simulink model "a_sim_1"  (R2020a)
settings: Solver=VariableStepAuto  StartTime=0.0  StopTime=10.0  RelTol=1e-3
values from neighbouring files (symbols this model uses):
  buffer = 0.0    (= 0)    [a_1.m]    (also in a_2.m; a_loss_function.m; full_model.m; part2.m)
  c_fi = 0.5    [a_1.m]    (also in a_2.m; a_loss_function.m; bank_and_economy.m = 0.25)
  gov = 0.5    [a_1.m]    (also in a_2.m; a_loss_function.m; bank_centralbank.m; full_model.m)
  hike = 0.0    (= 0)    [a_1.m]    (also in a_2.m = 0.01; a_loss_function.m; full_model.m; part2.m = 0.01)
  i_cb = 0.03    [a_1.m]    (also in a_2.m = 0.07; a_loss_function.m; full_model.m; part2.m = 0.1)
  i_diff = 0.025    [a_1.m]    (also in a_2.m; a_loss_function.m; bank_and_economy.m = 0.02; full_model.m)
  i_k = 0.06    [a_1.m]    (also in a_loss_function.m = 0.04; bank_and_economy.m = 0.04; full_model.m = 0.04)
  K_p = 15    [a_1.m]    (also in a_2.m; a_loss_function.m; bank_and_economy.m = 0.5; bank_centralbank.m)
  lambda = 0.002    [a_1.m]    (also in a_2.m; a_loss_function.m; bank_and_economy.m; bank_centralbank.m)
  lambda_k = 0.005    [a_1.m]    (also in a_2.m; a_loss_function.m; full_model.m; part2.m)
  R = 1    [a_1.m]    (also in a_2.m; a_loss_function.m; bank_and_economy.m; bank_centralbank.m)
  r_k = 0.1    [a_1.m]    (also in a_2.m; a_loss_function.m; bank_and_economy.m; full_model.m)
  rate = 0.1    [a_1.m]    (also in a_2.m; a_loss_function.m; bank_and_economy.m; bank_centralbank.m)
  s_k = 0.25    [a_1.m]    (also in a_2.m; bank_and_economy.m; part2.m = 0.2; part_1.m = 0.2)
  sigma = 0.28    [a_1.m]    (also in a_2.m; a_loss_function.m; bank_and_economy.m; bank_centralbank.m)
  T_f = 0.5    [a_1.m]    (also in a_2.m; a_loss_function.m; bank_and_economy.m; bank_centralbank.m)
  T_g = 1    [a_1.m]    (also in a_2.m; a_loss_function.m; bank_and_economy.m; bank_centralbank.m)
  T_h = 0.1    [a_1.m]    (also in a_2.m; a_loss_function.m; bank_and_economy.m; bank_centralbank.m)
  T_i = 8    [a_1.m]    (also in a_2.m; a_loss_function.m; bank_and_economy.m; bank_centralbank.m)
  T_k = 0.1    [a_1.m]    (also in a_2.m; a_loss_function.m; bank_and_economy.m = 0.25; economy.m = 1)
  tx = 0.3    [a_1.m]    (also in a_2.m; a_loss_function.m; bank_and_economy.m = 0.5; bank_centralbank.m = 0.25)
settings Model: Creator=erlended  LastModifiedBy=erlended

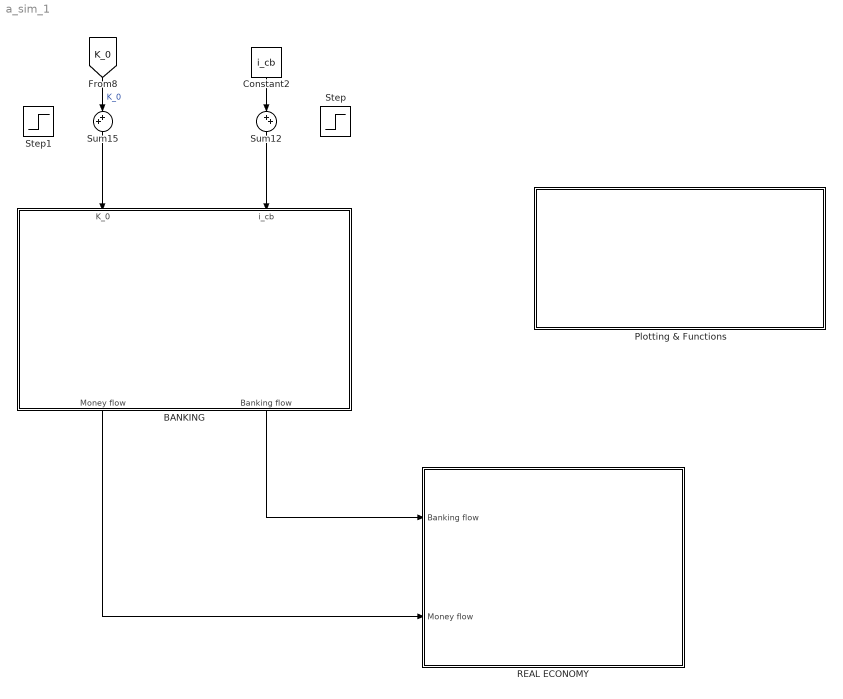
== system a_sim_1 ==
  BANKING : Subsystem
  Constant2 : Constant  Value=i_cb
  Plotting & Functions : Subsystem
  REAL ECONOMY : Subsystem
  Step : Step  Time=10  After=hike  SampleTime=0
  Step1 : Step  Time=10  After=buffer  SampleTime=0
  Sum12 : Sum  Inputs=|++
  Sum15 : Sum  Inputs=++|
  wires:
  Constant2/1 -> Sum12/1
  [K_0] -> Sum15/2  "K_0"
  BANKING/2(Banking flow) -> REAL ECONOMY/1(Banking flow)
  Sum12/1 -> BANKING/2(i_cb)
  BANKING/1(Money flow) -> REAL ECONOMY/2(Money flow)
  Sum15/1 -> BANKING/1(K_0)

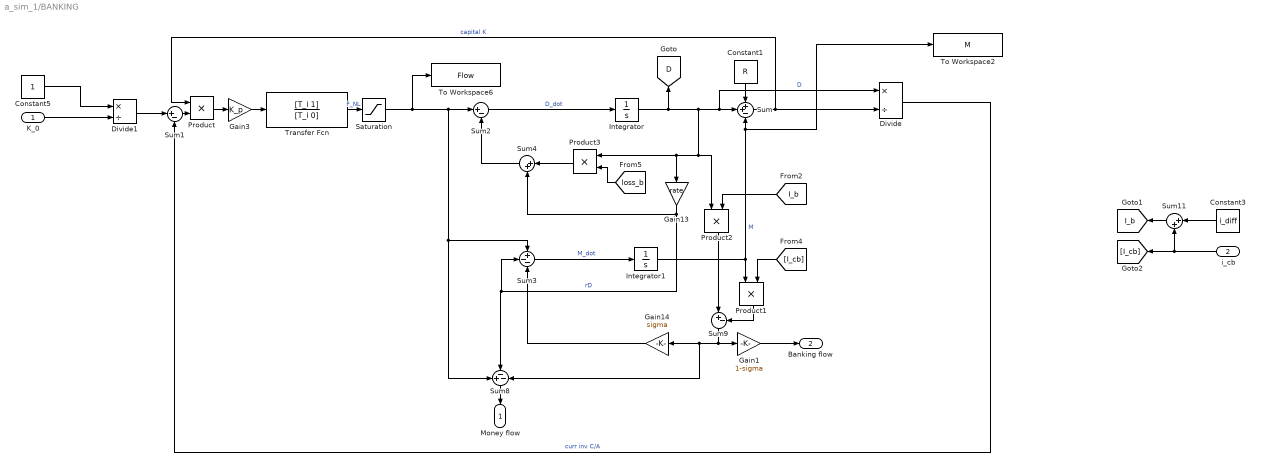
== system a_sim_1/BANKING ==
  K_0 : Inport
  i_cb : Inport  Port=2
  Constant1 : Constant  Value=R
  Constant3 : Constant  Value=i_diff
  Constant5 : Constant
  Divide : Product  Inputs=*/
  Divide1 : Product  Inputs=*/
  Gain1 : Gain  Gain=1-sigma
  Gain13 : Gain  Gain=rate
  Gain14 : Gain  Gain=sigma
  Gain3 : Gain  Gain=K_p
  Integrator : Integrator
  Integrator1 : Integrator
  Product{,1..3} (4 alike) : Product
  Saturation : Saturate  UpperLimit=100  LowerLimit=0
  Sum : Sum  Inputs=++-
  Sum1 : Sum  Inputs=|+-
  Sum11 : Sum  Inputs=|++
  Sum2 : Sum  Inputs=|+-
  Sum3 : Sum  Inputs=+--
  Sum4 : Sum  Inputs=|++
  Sum8 : Sum  Inputs=+--
  Sum9 : Sum  Inputs=|+-
  To Workspace2 : ToWorkspace  VariableName=M  SaveFormat=Timeseries  SampleTime=-1
  To Workspace6 : ToWorkspace  VariableName=Flow  SaveFormat=Timeseries  SampleTime=-1
  Transfer Fcn : TransferFcn  Numerator=[T_i 1]  Denominator=[T_i 0]
  Money flow : Outport
  Banking flow : Outport  Port=2
  tag scope: D=global, I_b=global
  wires:
  Product/1 -> Gain3/1
  Integrator/1 -> Sum/2, Divide/1, Product3/1, Gain13/1, Product2/1, [D]  "D"
  Sum8/1 -> Money flow/1
  Integrator1/1 -> To Workspace2/1, Sum/3, Product1/1  "M"
  Saturation/1 -> Sum2/1, Sum3/1, Sum8/1, To Workspace6/1
  Transfer Fcn/1 -> Saturation/1  "F_NL"
  Sum/1 -> Product/1, Divide/2  "capital K"
  Sum4/1 -> Sum2/2
  Gain13/1 -> Sum4/2, Sum8/2, Sum3/2  "rD"
  Sum9/1 -> Gain1/1, Sum8/3, Gain14/1
  Sum2/1 -> Integrator/1  "D_dot"
  Constant3/1 -> Sum11/1
  Gain3/1 -> Transfer Fcn/1
  Constant1/1 -> Sum/1
  Divide/1 -> Sum1/2  "curr inv C/A"
  Sum1/1 -> Product/2
  Sum3/1 -> Integrator1/1  "M_dot"
  Product2/1 -> Sum9/1
  Product1/1 -> Sum9/2
  Constant5/1 -> Divide1/1
  i_cb/1 -> [I_cb], Sum11/2
  Divide1/1 -> Sum1/1
  Gain14/1 -> Sum3/3
  Gain1/1 -> Banking flow/1
  K_0/1 -> Divide1/2
  Sum11/1 -> [I_b]
  [I_b] -> Product2/2
  [I_cb] -> Product1/2
  Product3/1 -> Sum4/1
  [loss_b] -> Product3/2

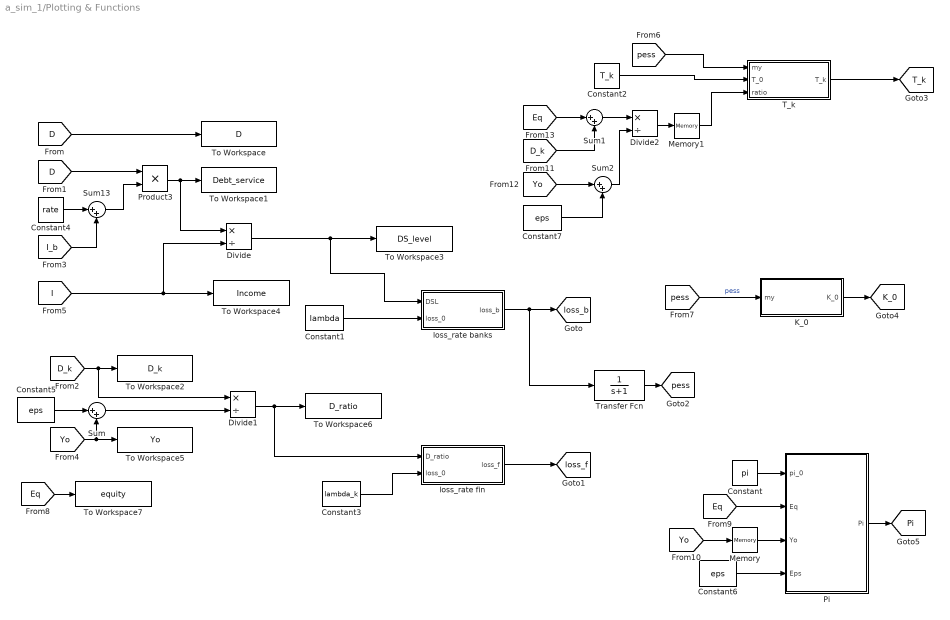
== system a_sim_1/Plotting & Functions ==
  Constant : Constant  Value=pi
  Constant1 : Constant  Value=lambda
  Constant2 : Constant  Value=T_k
  Constant3 : Constant  Value=lambda_k
  Constant4 : Constant  Value=rate
  Constant5 : Constant  Value=eps
  Constant6 : Constant  Value=eps
  Constant7 : Constant  Value=eps
  Divide : Product  Inputs=*/
  Divide1 : Product  Inputs=*/
  Divide2 : Product  Inputs=*/
  K_0 : MATLAB Function  TreatAsAtomicUnit=on
  Memory : Memory
  Memory1 : Memory
  Pi : MATLAB Function  TreatAsAtomicUnit=on
  Product3 : Product
  Sum{,1..2,13} (4 alike) : Sum  Inputs=|++
  T_k : MATLAB Function  TreatAsAtomicUnit=on
  To Workspace : ToWorkspace  VariableName=D  SaveFormat=Timeseries  SampleTime=-1
  To Workspace1 : ToWorkspace  VariableName=Debt_service  SaveFormat=Timeseries  SampleTime=-1
  To Workspace2 : ToWorkspace  VariableName=D_k  SaveFormat=Timeseries  SampleTime=-1
  To Workspace3 : ToWorkspace  VariableName=DS_level  SaveFormat=Timeseries  SampleTime=-1
  To Workspace4 : ToWorkspace  VariableName=Income  SaveFormat=Timeseries  SampleTime=-1
  To Workspace5 : ToWorkspace  VariableName=Yo  SaveFormat=Timeseries  SampleTime=-1
  To Workspace6 : ToWorkspace  VariableName=D_ratio  SaveFormat=Timeseries  SampleTime=-1
  To Workspace7 : ToWorkspace  VariableName=equity  SaveFormat=Timeseries  SampleTime=-1
  Transfer Fcn : TransferFcn  Denominator=[1 1]
  loss_rate banks : MATLAB Function  TreatAsAtomicUnit=on
  loss_rate fin : MATLAB Function  TreatAsAtomicUnit=on
  tag scope: K_0=global, Pi=global, T_k=global, loss_b=global, loss_f=global, pess=global
  wires:
  Divide/1 -> loss_rate banks/1(DSL), To Workspace3/1
  Constant3/1 -> loss_rate fin/2(loss_0)
  Sum/1 -> Divide1/2
  Divide1/1 -> loss_rate fin/1(D_ratio), To Workspace6/1
  Constant5/1 -> Sum/1
  Constant1/1 -> loss_rate banks/2(loss_0)
  [D_k] -> To Workspace2/1, Divide1/1
  [I] -> Divide/2, To Workspace4/1
  Constant4/1 -> Sum13/1
  [D] -> Product3/1
  [I_b] -> Sum13/2
  [D] -> To Workspace/1
  Product3/1 -> Divide/1, To Workspace1/1
  [Yo] -> Sum/2, To Workspace5/1
  Sum13/1 -> Product3/2
  loss_rate fin/1(loss_f) -> [loss_f]
  Transfer Fcn/1 -> [pess]
  Constant2/1 -> T_k/2(T_0)
  [pess] -> T_k/1(my)
  T_k/1(T_k) -> [T_k]
  [pess] -> K_0/1(my)  "pess"
  K_0/1(K_0) -> [K_0]
  loss_rate banks/1(loss_b) -> Transfer Fcn/1, [loss_b]
  Constant/1 -> Pi/1(pi_0)
  [Eq] -> To Workspace7/1
  [Eq] -> Pi/2(Eq)
  [Yo] -> Memory/1
  Pi/1(Pi) -> [Pi]
  Constant6/1 -> Pi/4(Eps)
  Memory/1 -> Pi/3(Yo)
  [Eq] -> Sum1/1
  [D_k] -> Sum1/2
  Sum1/1 -> Divide2/1
  Divide2/1 -> Memory1/1
  [Yo] -> Sum2/1
  Sum2/1 -> Divide2/2
  Constant7/1 -> Sum2/2
  Memory1/1 -> T_k/3(ratio)

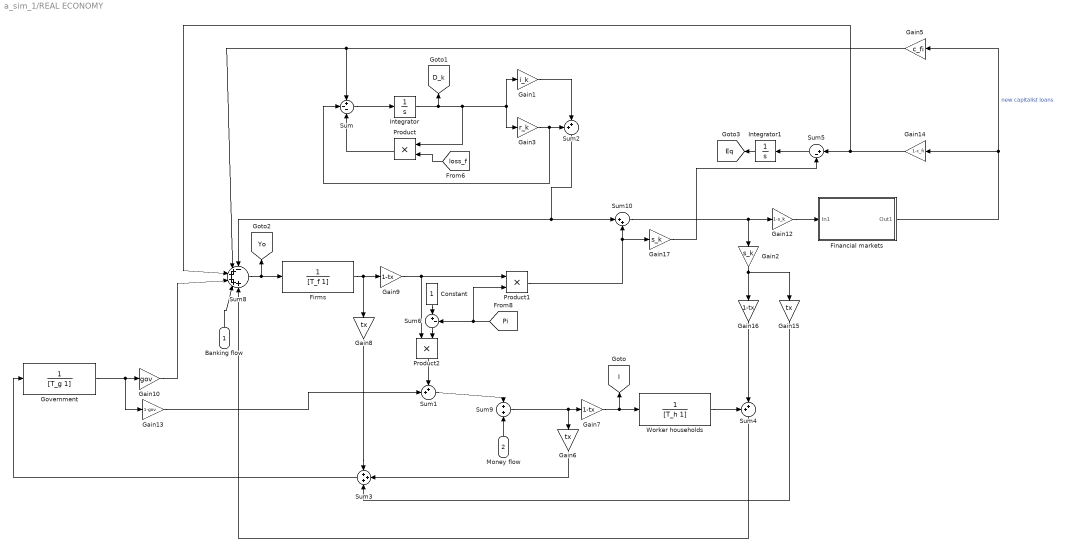
== system a_sim_1/REAL ECONOMY ==
  Banking flow : Inport
  Money flow : Inport  Port=2
  Constant : Constant
  Financial markets : Subsystem
  Firms : TransferFcn  Denominator=[T_f 1]
  Gain1 : Gain  Gain=i_k
  Gain10 : Gain  Gain=gov
  Gain12 : Gain  Gain=1-s_k
  Gain13 : Gain  Gain=1-gov
  Gain14 : Gain  Gain=1-c_fi
  Gain15 : Gain  Gain=tx
  Gain16 : Gain  Gain=1-tx
  Gain17 : Gain  Gain=s_k
  Gain2 : Gain  Gain=s_k
  Gain3 : Gain  Gain=r_k
  Gain5 : Gain  Gain=c_fi
  Gain6 : Gain  Gain=tx
  Gain7 : Gain  Gain=1-tx
  Gain8 : Gain  Gain=tx
  Gain9 : Gain  Gain=1-tx
  Government : TransferFcn  Denominator=[T_g 1]
  Integrator : Integrator
  Integrator1 : Integrator
  Product : Product
  Product1 : Product
  Product2 : Product
  Sum : Sum  Inputs=+--
  Sum1 : Sum  Inputs=++|
  Sum10 : Sum  Inputs=|++
  Sum2 : Sum  Inputs=++|
  Sum3 : Sum  Inputs=+++
  Sum4 : Sum  Inputs=++|
  Sum5 : Sum  Inputs=|+-
  Sum6 : Sum  Inputs=|+-
  Sum8 : Sum  Inputs=-+++++
  Sum9 : Sum
  Worker households : TransferFcn  Denominator=[T_h 1]
  tag scope: D_k=global, Eq=global, I=global, Yo=global
  wires:
  Gain1/1 -> Sum2/2
  Sum8/1 -> [Yo], Firms/1
  Integrator/1 -> [D_k], Product/1, Gain1/1, Gain3/1
  Sum2/1 -> Sum10/1, Sum8/1
  Gain3/1 -> Sum/2, Sum2/1
  Sum/1 -> Integrator/1
  Product/1 -> Sum/3
  Product1/1 -> Sum10/2, Gain17/1
  Sum9/1 -> Gain7/1, Gain6/1
  Money flow/1 -> Sum9/2
  Firms/1 -> Gain8/1, Gain9/1
  Sum3/1 -> Government/1
  Gain7/1 -> [I], Worker households/1
  Gain8/1 -> Sum3/1
  Gain6/1 -> Sum3/2
  Government/1 -> Gain13/1, Gain10/1
  Product2/1 -> Sum1/1
  Sum1/1 -> Sum9/1
  Gain13/1 -> Sum1/2
  Banking flow/1 -> Sum8/5
  Gain10/1 -> Sum8/4
  [loss_f] -> Product/2
  Gain12/1 -> Financial markets/1(In1)
  Gain14/1 -> Sum5/1, Sum8/3
  Financial markets/1(Out1) -> Gain5/1, Gain14/1  "new capitalist loans"
  Worker households/1 -> Sum4/1
  Sum4/1 -> Sum8/6
  Sum10/1 -> Gain12/1, Gain2/1
  Gain2/1 -> Gain15/1, Gain16/1
  Gain15/1 -> Sum3/3
  Gain16/1 -> Sum4/2
  Gain5/1 -> Sum8/2, Sum/1
  Sum5/1 -> Integrator1/1
  Gain17/1 -> Sum5/2
  Integrator1/1 -> [Eq]
  [Pi] -> Sum6/2, Product1/2
  Gain9/1 -> Product2/1, Product1/1
  Sum6/1 -> Product2/2
  Constant/1 -> Sum6/1

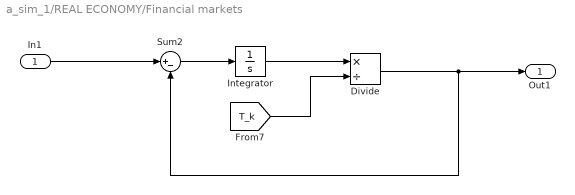
== system a_sim_1/REAL ECONOMY/Financial markets ==
  In1 : Inport
  Divide : Product  Inputs=*/
  Integrator : Integrator
  Sum2 : Sum  Inputs=|+-
  Out1 : Outport
  wires:
  In1/1 -> Sum2/1
  Sum2/1 -> Integrator/1
  Divide/1 -> Out1/1, Sum2/2
  Integrator/1 -> Divide/1
  [T_k] -> Divide/2

== matlab function a_sim_1/Plotting & Functions/loss_rate banks ==
  data: DSL input; loss_b output; loss_0 input
function loss_b = fcn(DSL,loss_0)

loss_b = 0.1*(DSL)^6+loss_0;

%if loss_b > 0.01
%    loss_b = 0.01;
%end

== matlab function a_sim_1/Plotting & Functions/K_0 ==
  data: my input; K_0 output
function K_0 = fcn(my)

%K_0 = 0.078+1*my;
K_0 = 0.08;

== matlab function a_sim_1/Plotting & Functions/loss_rate fin ==
  data: D_ratio input; loss_f output; loss_0 input
function loss_f = fcn(D_ratio,loss_0)

loss_f = 0.001*(D_ratio/1.8)^4+loss_0;

== matlab function a_sim_1/Plotting & Functions/T_k ==
  data: my input; T_k output; T_0 input; ratio input
function T_k = fcn(my,T_0, ratio)

%T_k = 0.55*(0.998+400*my)*T_0;
T_k = 0.03*(ratio)^2+2*my+T_0;

== matlab function a_sim_1/Plotting & Functions/Pi ==
  data: pi_0 input; Pi output; Eq input; Yo input; Eps input
function Pi = fcn(pi_0, Eq, Yo, Eps)

Pi = 0.1*Eq/(Yo+Eps)+pi_0;
if Pi > 0.6
    Pi = 0.6; 
end
